simulink model "pid_lqr_demo"  (R2019b)
settings: Solver=ode45  StartTime=0  StopTime=38  FixedStep=0.002  RelTol=1e-3  AbsTol=1e-6
libraries: Solver_SF x1, simulink x1
settings Model: ExtModeTrigMode=oneshot  ExtModeArmWhenConnect=off  Creator=ywata  LastModifiedBy=saxijing
settings SolverCC: AutoScaleAbsTol=off
settings DataIOCC: SaveFormat=Array  SignalLoggingSaveFormat=ModelDataLogs  ReturnWorkspaceOutputs=off  SignalLoggingName=sigsOut
settings OptimizationCC: BlockReduction=off  BooleanDataType=off  LifeSpan=inf
settings DebuggingCC: SaveWithParameterizedLinksMsg=none  UnderspecifiedInitializationDetection=Classic  MergeDetectMultiDrivingBlocksExec=none  SignalResolutionControl=TryResolveAllWithWarning  MultiTaskDSMMsg=warning  MultiTaskCondExecSysMsg=none  FcnCallInpInsideContextMsg=warning  StateNameClashWarn=warning  SFUnexpectedBacktrackingDiag=warning  SFNoUnconditionalDefaultTransitionDiag=warning  ArithmeticOperatorsInVariantConditions=warning
settings HardwareCC: ProdBitPerPointer=32  ProdBitPerSizeT=32  ProdBitPerPtrDiffT=32  ProdLargestAtomicFloat=None  ProdIntDivRoundTo=Undefined  ProdEndianess=Unspecified  ProdWordSize=32  ProdHWDeviceType=32-bit Generic  TargetUnknown=on
settings ModelReferenceCC: PropagateSignalLabelsOutOfModel=off
settings SFSimCC: SimUseLocalCustomCode=off  CustomCodeUndefinedFunction=UseInterfaceOnly
settings RTWCC: TemplateMakefile=grt_vc.tmf  RTWUseLocalCustomCode=off
settings CodeAppCC: StateflowObjectComments=on
settings GRTTargetCC: TargetFcnLib=ansi_tfl_tmw.mat  TargetLangStandard=C89/C90 (ANSI)  CombineOutputUpdateFcns=off  GRTInterface=on
settings ConfigComp: CovMetricSettings=dw  CovHtmlReporting=on  CovSaveCumulativeToWorkspaceVar=on  CovSaveSingleToWorkspaceVar=on  CovExternalEMLEnable=off

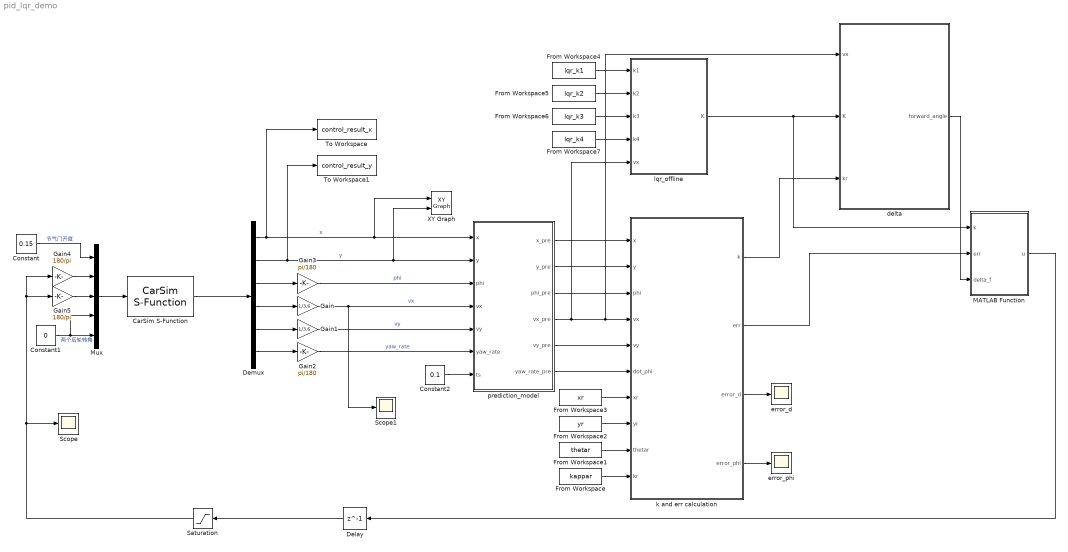
== system pid_lqr_demo ==
  CarSim S-Function : Solver_SF/CarSim S-Function  Priority=1  VehicleCode=i_i  SIMFILE=simfile.sim
  Constant : Constant  Value=0.15
  Constant1 : Constant  Value=0
  Constant2 : Constant  Value=0.1
  Delay : Delay  DelayLength=1
  Demux : Demux  Outputs=6
  From Workspace : FromWorkspace  VariableName=kappar  SampleTime=0
  From Workspace1 : FromWorkspace  VariableName=thetar  SampleTime=0
  From Workspace2 : FromWorkspace  VariableName=yr  SampleTime=0
  From Workspace3 : FromWorkspace  VariableName=xr  SampleTime=0
  From Workspace4 : FromWorkspace  VariableName=lqr_k1  SampleTime=0
  From Workspace5 : FromWorkspace  VariableName=lqr_k2  SampleTime=0
  From Workspace6 : FromWorkspace  VariableName=lqr_k3  SampleTime=0
  From Workspace7 : FromWorkspace  VariableName=lqr_k4  SampleTime=0
  Gain : Gain  Gain=1/3.6
  Gain1 : Gain  Gain=1/3.6
  Gain2 : Gain  Gain=pi/180
  Gain3 : Gain  Gain=pi/180
  Gain4 : Gain  Gain=180/pi
  Gain5 : Gain  Gain=180/pi
  MATLAB Function : MATLAB Function  TreatAsAtomicUnit=on
  Mux : Mux  Inputs=5
  Saturation : Saturate  UpperLimit=0.69  LowerLimit=-0.69
  Scope : Scope
  Scope1 : Scope
  To Workspace : ToWorkspace  VariableName=control_result_x  SampleTime=-1
  To Workspace1 : ToWorkspace  VariableName=control_result_y  SampleTime=-1
  XY Graph : simulink/Sinks/XY Graph  xmin=-20  xmax=80  ymin=-10  ymax=60  st=-1
  delta : MATLAB Function  TreatAsAtomicUnit=on
  error_d : Scope
  error_phi : Scope
  k and err calculation : MATLAB Function  TreatAsAtomicUnit=on
  lqr_offline : MATLAB Function  TreatAsAtomicUnit=on
  prediction_model : MATLAB Function  TreatAsAtomicUnit=on
  wires:
  Mux/1 -> CarSim S-Function/1
  CarSim S-Function/1 -> Demux/1
  Demux/4 -> Gain/1
  Demux/5 -> Gain1/1
  Demux/6 -> Gain2/1
  Demux/2 -> To Workspace1/1, XY Graph/2, prediction_model/2(y)  "y"
  Demux/1 -> To Workspace/1, XY Graph/1, prediction_model/1(x)  "x"
  Gain/1 -> Scope1/1, prediction_model/4(vx)  "vx"
  Gain1/1 -> prediction_model/5(vy)  "vy"
  Gain2/1 -> prediction_model/6(yaw_rate)  "yaw_rate"
  Demux/3 -> Gain3/1
  Gain3/1 -> prediction_model/3(phi)  "phi"
  Constant2/1 -> prediction_model/7(ts)
  prediction_model/6(yaw_rate_pre) -> k and err calculation/6(dot_phi)
  prediction_model/5(vy_pre) -> k and err calculation/5(vy)
  prediction_model/4(vx_pre) -> lqr_offline/5(vx), delta/1(vx), k and err calculation/4(vx)
  prediction_model/2(y_pre) -> k and err calculation/2(y)
  prediction_model/1(x_pre) -> k and err calculation/1(x)
  prediction_model/3(phi_pre) -> k and err calculation/3(phi)
  From Workspace3/1 -> k and err calculation/7(xr)
  From Workspace2/1 -> k and err calculation/8(yr)
  From Workspace1/1 -> k and err calculation/9(thetar)
  From Workspace/1 -> k and err calculation/10(kr)
  From Workspace7/1 -> lqr_offline/4(k4)
  From Workspace6/1 -> lqr_offline/3(k3)
  From Workspace5/1 -> lqr_offline/2(k2)
  From Workspace4/1 -> lqr_offline/1(k1)
  lqr_offline/1(K) -> MATLAB Function/1(k), delta/2(K)
  k and err calculation/1(k) -> delta/3(kr)
  k and err calculation/2(err) -> MATLAB Function/2(err)
  delta/1(forward_angle) -> MATLAB Function/3(delta_f)
  MATLAB Function/1(u) -> Delay/1
  Gain4/1 -> Mux/2
  Gain5/1 -> Mux/3
  Delay/1 -> Saturation/1
  Constant/1 -> Mux/1  "节气门开度"
  Constant1/1 -> Mux/4, Mux/5  "两个后轮转角"
  Saturation/1 -> Gain5/1, Gain4/1, Scope/1
  k and err calculation/3(error_d) -> error_d/1
  k and err calculation/4(error_phi) -> error_phi/1

== matlab function pid_lqr_demo/k and err calculation ==
  data: x input; k output; y input; phi input; vx input; vy input; dot_phi input; xr input; yr input; thetar input; kr input; err output; error_d output; error_phi output
function [k,err,error_d,error_phi]=fcn(x,y,phi,vx,vy,dot_phi,xr,yr,thetar,kr)
    len=length(xr);
    d_min=(x-xr(1))^2+(y-yr(1))^2;
    match_id=1;
    for i=1:len
        d=(x-xr(i))^2+(y-yr(i))^2;
        if d<d_min
            d_min=d;
            match_id=i;
        end
    end
    tor=[cos(thetar(match_id)),sin(thetar(match_id))]';
    nor=[-sin(thetar(match_id)),cos(thetar(match_id))]';
    d_err=[x-xr(match_id),y-yr(match_id)]';
    error_d=nor'*d_err;
    error_s=tor'*d_err;
    projection_theta=thetar(match_id)+kr(match_id)*error_s;
    dot_error_d=vy*cos(phi-projection_theta)+vx*sin(phi-projection_theta);
    %suppose phi=sin phi,in case of 2*pi
    error_phi=sin(phi-projection_theta);
    dot_s=(vx*cos(phi-projection_theta)-vy*sin(phi-projection_theta))/(1-kr(match_id)*error_d);
    dot_error_phi=dot_phi-kr(match_id)*dot_s;
    k=kr(match_id);
    err=[error_d;dot_error_d;error_phi;dot_error_phi];
end

== matlab function pid_lqr_demo/prediction_model ==
  data: x input; x_pre output; y input; phi input; vx input; vy input; yaw_rate input; y_pre output; phi_pre output; vx_pre output; vy_pre output; yaw_rate_pre output; ts input
function [x_pre,y_pre,phi_pre,vx_pre,vy_pre,yaw_rate_pre]=fcn(x,y,phi,vx,vy,yaw_rate,ts)
    x_pre=x+vx*ts*cos(phi)-vy*ts*sin(phi);
    y_pre=y+vy*ts*cos(phi)+vx*ts*sin(phi);
    phi_pre=phi+yaw_rate*ts;
    vx_pre=vx;
    vy_pre=vy;
    yaw_rate_pre=yaw_rate;
end

== matlab function pid_lqr_demo/lqr_offline ==
  data: k1 input; K output; k2 input; k3 input; k4 input; vx input
function K  = fcn(k1,k2,k3,k4,vx)
    if abs(vx)<0.01
        K=[0,0,0,0]
    else
        index=round(vx/0.01);
        K=[k1(index),k2(index),k3(index),k4(index)];
    end
end

== matlab function pid_lqr_demo/delta ==
  data: vx input; forward_angle output; K input; kr input
function forward_angle = fcn(vx,K,kr)
    cf=-110000;
    cr=cf;
    m=1270+71*2;
    a=1.015;
    b=2.910-1.015;
    Iz=1536.7;
    forward_angle=kr*(a+b-b*K(3)-(m*vx*vx/(a+b))*(b/cf+a*K(3)/cr-a/cr));
end

== matlab function pid_lqr_demo/MATLAB Function ==
  data: k input; u output; err input; delta_f input
function u = fcn(k,err,delta_f)
    u=-k*err+delta_f;
end
